simulink model "Rectifier"  (Simulink 7.1)
settings: Solver=ode45  StartTime=0.0  StopTime=.5  RelTol=1e-3
libraries: simulink x1
settings Model: Creator=Smrit  LastModifiedBy=Smrit

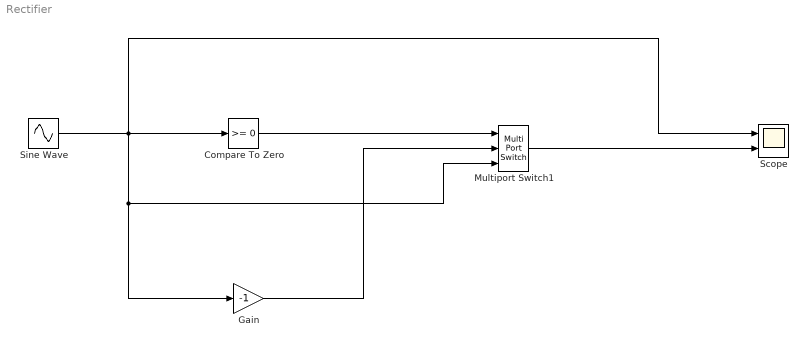
== system Rectifier ==
  Compare To Zero : simulink/Logic and Bit Operations/Compare To Zero  SystemSampleTime=-1  relop=>=  LogicOutDataTypeMode=uint8  ZeroCross=off
  Gain : Gain  Gain=-1  ParameterDataType=sfix(16)  ParameterScaling=2^0  OutDataType=sfix(16)  OutScaling=2^0
  Multiport Switch1 : MultiPortSwitch  Inputs=2  zeroidx=on  OutDataType=sfix(16)  OutScaling=2^0
  Scope : Scope  NumInputPorts=2
      settings: TimeRange=2  YMin=-5~-5  YMax=5~5
  Sine Wave : Sin  Amplitude=20  Frequency=25  SampleTime=0  VectorParams1D=off
  wires:
  Sine Wave/1 -> Compare To Zero/1, Multiport Switch1/3, Gain/1, Scope/1
  Compare To Zero/1 -> Multiport Switch1/1
  Multiport Switch1/1 -> Scope/2
  Gain/1 -> Multiport Switch1/2
